simulink model "P4_RaspberryModel_with_DT"  (R2025b)
settings: Solver=daessc  StartTime=0.0  StopTime=Inf  FixedStep=0.01  RelTol=1e-3
PreLoadFcn:
  | % Kalman Filter testing
  | m=0.370;
  | l=0.075; %0.079793%determined by pendulum experiment %former values 0.032, 0.035;
  | lm=l*m; %lm=0.032*0.377
  | r=0.0405;
  | rm=r*m; %rm=0.0405*0.377
  | K=1;
  | 
  | tem=0.2 %initial guess
  | eta=2*lm+rm+(2*m*l^2/r);
  | 
  | A31=(lm+rm)/(tem*eta);
  | A32=9.81*lm/(r*eta);
  | A=[0 1 0 0; 0 -1/tem, 0, 0; 0, 0, 0, 1; 0 A31, A32, 0];
  | B=[0; 1/tem;0;-A31];
model workspace (MAT data in the model file):
  Amp = 1
undefined symbols (not defined in the file): anglerate, DiscIntNeverNeededParam, motor_left, motor_param, motor_right, PosEnc, VelEnc
libraries: simulink x19, raspberrypiCommlib x7, dspstat3 x6, slpidlib x3, sm_lib x3, raspberrypiNetworklib x2, svdutilitieslib x2, SigiLib x2, robotcorelib x1, mspfiltlib x1, nesl_utility x1
(part 1 of 2)
settings Model: SimulationMode=external  NumberOfSteps=10  ExtModeTrigDuration=2  Creator=resjoehr  LastModifiedBy=resjoehr
settings SolverCC: AlgebraicLoopSolver=TrustRegion  PositivePriorityOrder=on
settings OptimizationCC: EnhancedBackFolding=on  PassReuseOutputArgsAs=Individual arguments  ZeroExternalMemoryAtStartup=off  ZeroInternalMemoryAtStartup=off  MaxStackSize=200000  OptimizeBlockOrder=speed  DifferentSizesBufferReuse=on  OptimizationCustomize=off  EfficientTunableParamExpr=on
settings DebuggingCC: ParameterTunabilityLossMsg=error  UnconnectedInputMsg=warning  UnconnectedOutputMsg=warning  UnconnectedLineMsg=warning
settings HardwareCC: ProdBitPerPointer=32.0  ProdBitPerSizeT=32.0  ProdBitPerPtrDiffT=32.0  ProdLargestAtomicInteger=Long  ProdLargestAtomicFloat=Double  ProdWordSize=32.0  ProdLongLongMode=on  ProdHWDeviceType=ARM Compatible->ARM Cortex-A (32-bit)
settings ModelReferenceCC: EnableRefExpFcnMdlSchedulingChecks=on
settings RTWCC: SystemTargetFile=ert.tlc  HardwareBoard=Raspberry Pi  TLCOptions="-aInlineSetEventsForThisBaseRateFcn=TLC_FALSE -aSuppressMultiTaskScheduler=TLC_FALSE  -aRateBasedStepFcn=0"  TemplateMakefile=ert_default_tmf  Toolchain=GNU GCC Embedded Linux  BuildConfiguration=Faster Runs  GPUComputeCapability=3.5  DLArmComputeVersion=19.05  Description=Embedded Coder
settings CodeAppCC: ForceParamTrailComments=on  IgnoreCustomStorageClasses=off  OperatorAnnotations=on  SimulinkDataObjDesc=on  SFDataObjDesc=on  InsertBlockDesc=on
settings ERTTargetCC: ExtModeTransport=2.0  ExtModeStaticAlloc=on  ExtModeMexFile=ext_xcp  ExtModeIntrfLevel=Level2 - Open  InlinedParameterPlacement=Hierarchical  DynamicArrayContainerType=coder::array  SupportVariableSizeSignals=on

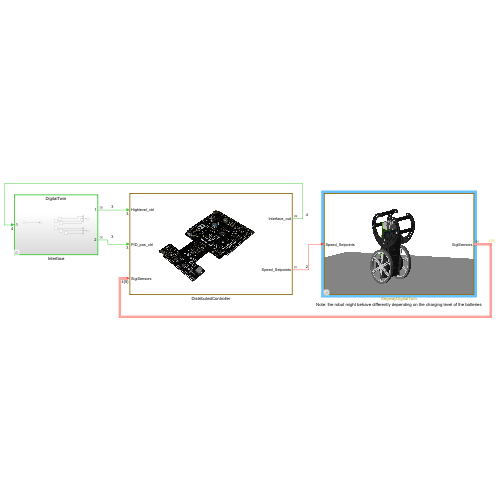
[thumbnail: Simulink's stored preview of the top-level diagram]
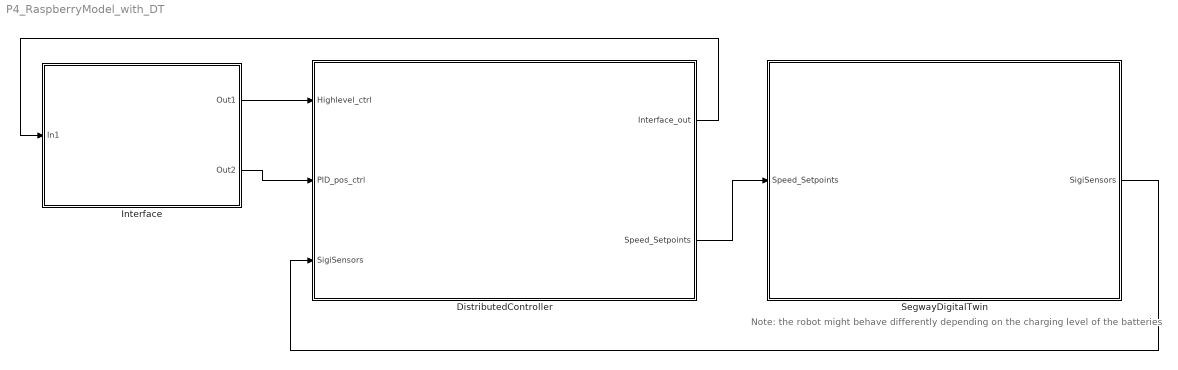
== system P4_RaspberryModel_with_DT ==
  note: Note: the robot might behave differently depending on the charging level of the batteries
  DistributedController : Subsystem
      mask Display: image('leonardo.jpg');
  Interface : Subsystem  Variant=on  VariantControlMode=sim codegen switching
  SegwayDigitalTwin : Subsystem  Variant=on  VariantControlMode=sim codegen switching  VariantControl=SegwayDigitalTwin
      mask Display: image('whole_sigi.jpg');
  wires:
  Interface/1(Out1) -> DistributedController/1(Highlevel_ctrl)
  Interface/2(Out2) -> DistributedController/2(PID_pos_ctrl)
  DistributedController/1(Interface_out) -> Interface/1(In1)
  DistributedController/2(Speed_Setpoints) -> SegwayDigitalTwin/1(Speed_Setpoints)
  SegwayDigitalTwin/1(SigiSensors) -> DistributedController/3(SigiSensors)

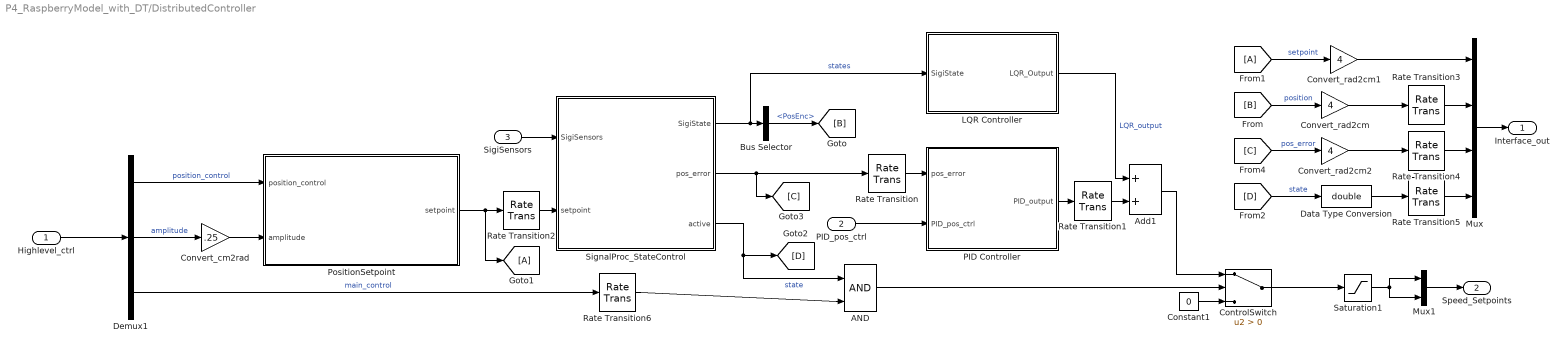
== system P4_RaspberryModel_with_DT/DistributedController ==
  Highlevel_ctrl : Inport  SampleTime=0.1
  PID_pos_ctrl : Inport  Port=2  SampleTime=0.1
  SigiSensors : Inport  Port=3  OutDataTypeStr=Bus: Sensors
  AND : Logic  IconShape=distinctive  AllPortsSameDT=off  OutDataTypeStr=boolean
  Add1 : Sum  OutDataTypeStr=double
  Bus Selector : BusSelector  OutputSignals=PosEnc
  Constant1 : Constant  Value=0  SampleTime=0.01
  ControlSwitch : Switch  Criteria=u2 > Threshold  SaturateOnIntegerOverflow=off  InputSameDT=off
  Convert_cm2rad : Gain  Gain=.25
  Convert_rad2cm : Gain  Gain=4
  Convert_rad2cm1 : Gain  Gain=4
  Convert_rad2cm2 : Gain  Gain=4
  Data Type Conversion : DataTypeConversion  OutDataTypeStr=double  SaturateOnIntegerOverflow=off  RndMeth=Floor
  Demux1 : Demux  Outputs=3
  From1 : From
  Goto1 : Goto
  LQR Controller : Subsystem
  Mux : Mux
  Mux1 : Mux  Inputs=2
  PID Controller : Subsystem
  PositionSetpoint : Subsystem
  Rate Transition{,3..5} (4 alike) : RateTransition  OutPortSampleTime=0.1
  Rate Transition1 : RateTransition  OutPortSampleTime=0.01
  Rate Transition2 : RateTransition  OutPortSampleTime=0.01
  Rate Transition6 : RateTransition  OutPortSampleTime=0.01
  Saturation1 : Saturate  UpperLimit=30  LowerLimit=-30
  SignalProc_StateControl : Subsystem  Variant=on  VariantControlMode=label  LabelModeActiveChoice=SensorFusion
  Interface_out : Outport  SampleTime=0.1
  Speed_Setpoints : Outport  Port=2
  wires:
  Highlevel_ctrl/1 -> Demux1/1
  Demux1/3 -> Rate Transition6/1  "main_control"
  Constant1/1 -> ControlSwitch/3
  AND/1 -> ControlSwitch/2
  Mux1/1 -> Speed_Setpoints/1
  Add1/1 -> ControlSwitch/1
  PID Controller/1(PID_output) -> Rate Transition1/1
  SignalProc_StateControl/3(active) -> [D], AND/1  "state"
  SignalProc_StateControl/1(SigiState) -> Bus Selector/1, LQR Controller/1(SigiState)  "states"
  SigiSensors/1 -> SignalProc_StateControl/1(SigiSensors)
  PID_pos_ctrl/1 -> PID Controller/2(PID_pos_ctrl)
  ControlSwitch/1 -> Saturation1/1
  [C] -> Convert_rad2cm2/1  "pos_error"
  [B] -> Convert_rad2cm/1  "position"
  Mux/1 -> Interface_out/1
  From1/1 -> Convert_rad2cm1/1  "setpoint"
  [D] -> Data Type Conversion/1  "state"
  SignalProc_StateControl/2(pos_error) -> [C], Rate Transition/1
  PositionSetpoint/1(setpoint) -> Goto1/1, Rate Transition2/1
  Demux1/1 -> PositionSetpoint/1(position_control)  "position_control"
  Demux1/2 -> Convert_cm2rad/1  "amplitude"
  Data Type Conversion/1 -> Rate Transition5/1
  Saturation1/1 -> Mux1/1, Mux1/2
  Convert_cm2rad/1 -> PositionSetpoint/2(amplitude)
  Convert_rad2cm/1 -> Rate Transition3/1
  Convert_rad2cm2/1 -> Rate Transition4/1
  Bus Selector/1 -> [B]  "<PosEnc>"
  LQR Controller/1(LQR_Output) -> Add1/1  "LQR_output"
  Rate Transition/1 -> PID Controller/1(pos_error)
  Rate Transition1/1 -> Add1/2
  Convert_rad2cm1/1 -> Mux/1
  Rate Transition3/1 -> Mux/2
  Rate Transition4/1 -> Mux/3
  Rate Transition5/1 -> Mux/4
  Rate Transition6/1 -> AND/2
  Rate Transition2/1 -> SignalProc_StateControl/2(setpoint)

== system P4_RaspberryModel_with_DT/Interface ==
  note: 1) Add Subsystem or Model blocks as valid variant choices.
      | 2) You cannot connect blocks at this level. At simulation, connectivity is automatically
      | determined, based on the active variant and port name matching.
  In1 : Inport
  DigitalTwin : Subsystem  VariantControl=(sim)
  Websocket : Subsystem  VariantControl=(codegen)
  Out1 : Outport
  Out2 : Outport  Port=2

== system P4_RaspberryModel_with_DT/SegwayDigitalTwin ==
  Speed_Setpoints : Inport  OutDataTypeStr=double
  RaspberryImplementation : Subsystem  VariantControl=(codegen)
  SegwayDigitalTwin : Subsystem  VariantControl=(sim)
      mask Display: image('whole_sigi.jpg');
  SigiSensors : Outport  OutDataTypeStr=Bus: Sensors

== system P4_RaspberryModel_with_DT/DistributedController/LQR Controller ==
  SigiState : Inport  OutDataTypeStr=Bus: States
  Bus Selector : BusSelector  OutputSignals=PosEnc,VelEnc,angle,anglerate
  Constant : Constant  Value=1.43  SampleTime=0.01
  Constant1 : Constant  Value=28.6  SampleTime=0.01
  Constant2 : Constant  Value=1.925  SampleTime=0.01
  Gain : Gain  Gain=0
  Product : Product
  Product1 : Product
  Product2 : Product
  Sum : Sum  Inputs=++++
  LQR_Output : Outport
  wires:
  Bus Selector/1 -> Gain/1  "<PosEnc>"
  Sum/1 -> LQR_Output/1
  Bus Selector/4 -> Product2/1  "<anglerate>"
  Bus Selector/3 -> Product1/1  "<angle>"
  Constant/1 -> Product/2
  Constant1/1 -> Product1/2
  Constant2/1 -> Product2/2
  Product/1 -> Sum/2
  Product1/1 -> Sum/3
  Product2/1 -> Sum/4
  Gain/1 -> Sum/1
  SigiState/1 -> Bus Selector/1
  Bus Selector/2 -> Product/1  "<VelEnc>"

== system P4_RaspberryModel_with_DT/DistributedController/PID Controller ==
  pos_error : Inport
  PID_pos_ctrl : Inport  Port=2
  Demux2 : Demux  Outputs=3
  Filter : Constant  Value=10  SampleTime=0.1
  Gain : Gain  Gain=-1
  Gain1 : Gain  Gain=-1
  Gain2 : Gain  Gain=-1
  Position Controller1 : slpidlib/PID Controller  Controller=PID  Form=Parallel  TimeDomain=Discrete-time  UseExternalTs=off  SampleTime=0.1  IntegratorMethod=Forward Euler  FilterMethod=Forward Euler  ControllerParametersSource=external  P=-0.3  I=0  UseKiTs=off  D=0.1  UseExternalDerivativeSource=off  N=10  UseFilter=on  TunerSelectOption=Transfer Function Based (PID Tuner App)  InitialConditionSource=internal  InitialConditionForIntegrator=0  InitialConditionForFilter=0  DifferentiatorICPrevScaledInput=0  ExternalReset=none  TrackingMode=off  Kt=1  LimitOutput=on  SatLimitsSource=internal  UpperSaturationLimit=20  LowerSaturationLimit=-20  LinearizeAsGain=on  AntiWindupMode=none  Kb=1  LimitIntegrator=off  UpperIntegratorSaturationLimit=inf  LowerIntegratorSaturationLimit=-inf  POutMin=[]  POutMax=[]  IOutMin=[]  IOutMax=[]  DOutMin=[]  DOutMax=[]  NOutMin=[]  NOutMax=[]  SumOutMin=[]  SumOutMax=[]  SaturationOutMin=[]  SaturationOutMax=[]  PParamMin=[]  PParamMax=[]  IParamMin=[]  IParamMax=[]  DParamMin=[]  DParamMax=[]  NParamMin=[]  NParamMax=[]  KbParamMin=[]  KbParamMax=[]  KtParamMin=[]  KtParamMax=[]  KbOutMin=[]  KbOutMax=[]  KtOutMin=[]  KtOutMax=[]  IntegratorOutMin=[]  IntegratorOutMax=[]  FilterOutMin=[]  FilterOutMax=[]  SumI1OutMin=[]  SumI1OutMax=[]  SumI2OutMin=[]  SumI2OutMax=[]  SumI3OutMin=[]  SumI3OutMax=[]  SumI4OutMin=[]  SumI4OutMax=[]  SumDOutMin=[]  SumDOutMax=[]  DifferentiatorOutMin=[]  DifferentiatorOutMax=[]  FilterDiffOutCoefMin=[]  FilterDiffOutCoefMax=[]  ReciprocalOutMin=[]  ReciprocalOutMax=[]  SumDenOutMin=[]  SumDenOutMax=[]  SumNumOutMin=[]  SumNumOutMax=[]  DivideOutMin=[]  DivideOutMax=[]  UdiffTsProdOutMin=[]  UdiffTsProdOutMax=[]  NTsProdOutMin=[]  NTsProdOutMax=[]  UintegralTsProdOutMin=[]  UintegralTsProdOutMax=[]  UngainTsProdOutMin=[]  UngainTsProdOutMax=[]  ClampingZeroOutDataTypeStr=Inherit: Inherit via back propagation  ClampingZeroOutMin=[]  ClampingZeroOutMax=[]  FilterDenConstantOutDataTypeStr=Inherit: Inherit via back propagation  FilterDenConstantOutMin=[]  FilterDenConstantOutMax=[]  PCopyOutDataTypeStr=Inherit: Inherit via back propagation  PCopyOutMin=[]  PCopyOutMax=[]  NCopyOutDataTypeStr=Inherit: Inherit via back propagation  NCopyOutMin=[]  NCopyOutMax=[]  IntegratorContinuousStateAttributes=''  IntegratorStateMustResolveToSignalObject=off  IntegratorRTWStateStorageClass=Auto  FilterContinuousStateAttributes=''  FilterStateMustResolveToSignalObject=off  FilterRTWStateStorageClass=Auto  ParallelPVariant=ExternalParameters  IdealPVariant=Disabled  IVariant=ExternalParameters  DVariant=ExternalParameters  IntegratorVariant=Discrete  SatVariant=Enabled  AWVariant=Passthrough  PCopyVariant=Disabled  TRVariant=Disabled  FdbkBlocksVariant=Forward  IdealPFdbkVariant=Disabled  SatFdbkVariant=Disabled  DerivativeFilterVariant=ForwardEulerFilter  NVariant=ExternalParameters  NCopyVariant=Disabled  FilterICVariant=InternalICsFilter  IntegratorICVariant=InternalICs  ExternalResetVariant=Disabled  TRSumVariant=Passthrough  SumFdbkVariant=Disabled  SumVariant=Sum_PID  TsampFilterVariant=InternalTs  TsampNgainVariant=Passthrough  TsampIntegralVariant=Disabled_SignalSpec  ExternalSaturationOutDataTypeStr=Inherit: Same as second input  DerivativeSourceVariant=ErrorSignal  PreIntVariant=InternalPreInt
  PID_output : Outport
  wires:
  Demux2/1 -> Gain/1
  Gain2/1 -> Position Controller1/4
  Gain/1 -> Position Controller1/2
  Filter/1 -> Position Controller1/5
  Demux2/3 -> Gain2/1
  Gain1/1 -> Position Controller1/3
  Demux2/2 -> Gain1/1
  PID_pos_ctrl/1 -> Demux2/1
  pos_error/1 -> Position Controller1/1  "setpoint"
  Position Controller1/1 -> PID_output/1

== system P4_RaspberryModel_with_DT/DistributedController/PositionSetpoint ==
  note: Position Setpoint
  position_control : Inport
  amplitude : Inport  Port=2
  Add3 : Sum  Inputs=+-
  Gain : Gain  Gain=0
  Gain5 : Gain
  Product1 : Product  Inputs=3
  Pulse Generator1 : DiscretePulseGenerator  Period=200  PulseWidth=100  PhaseDelay=100  SampleTime=0.1
  setpoint : Outport
  wires:
  Product1/1 -> Gain5/1  "setpoint"
  Gain/1 -> Add3/2
  Gain5/1 -> Add3/1
  amplitude/1 -> Product1/2, Gain/1
  Pulse Generator1/1 -> Product1/3
  Add3/1 -> setpoint/1  "setpoint"
  position_control/1 -> Product1/1

== system P4_RaspberryModel_with_DT/DistributedController/SignalProc_StateControl ==
  note: 1) Add Subsystem or Model blocks as valid variant choices.
      | 2) You cannot connect blocks at this level. At simulation, connectivity is automatically
      | determined, based on the active variant and port name matching.
  SigiSensors : Inport  OutDataTypeStr=Bus: Sensors
  setpoint : Inport  Port=2
  ClassicalCalibration : Subsystem  VariantControl=ClassicalCalibration
  SensorFusion : Subsystem  VariantControl=SensorFusion
  SigiState : Outport  OutDataTypeStr=Bus: States
  pos_error : Outport  Port=2
  active : Outport  Port=3

== system P4_RaspberryModel_with_DT/Interface/DigitalTwin ==
  In1 : Inport  OutDataTypeStr=double
  Constant : Constant  Value=0  SampleTime=0.1
  Constant1 : Constant  Value=0  SampleTime=0.1
  Constant2 : Constant  Value=0.5  SampleTime=0.1
  Constant3 : Constant  SampleTime=0.1
  Constant4 : Constant  SampleTime=0.1
  Constant5 : Constant  Value=10  SampleTime=0.1
  Mux2 : Mux  Inputs=3
  Mux3 : Mux  Inputs=3
  Terminator : Terminator
  Out1 : Outport
  Out2 : Outport  Port=2
  wires:
  In1/1 -> Terminator/1
  Constant5/1 -> Mux2/2  "amplitude"
  Constant3/1 -> Mux2/3  "main control"
  Constant4/1 -> Mux2/1  "enable_pos_control"
  Mux2/1 -> Out1/1
  Constant2/1 -> Mux3/1  "p-gain"
  Mux3/1 -> Out2/1
  Constant1/1 -> Mux3/2  "i-gain"
  Constant/1 -> Mux3/3  "d-gain"

== system P4_RaspberryModel_with_DT/Interface/Websocket ==
  In1 : Inport
  Demux : Demux
  FromWebSocket : Subsystem
  Websocket publish : raspberrypiNetworklib/WebSocket publish  UniqueBlockID=webPub 1  IPAddress=192.168.43.245  Port=9000  NumberOfSignals=4  webSocketId=P4_RaspberryModel_with_DT/Interface/Websocket/Websocket_publish  BlockPlatform=RASPBERRYPI
  Out1 : Outport
  Out2 : Outport  Port=2
  wires:
  In1/1 -> Demux/1
  Demux/1 -> Websocket publish/1
  Demux/2 -> Websocket publish/2
  Demux/3 -> Websocket publish/3
  Demux/4 -> Websocket publish/4
  FromWebSocket/2(Out2) -> Out2/1
  FromWebSocket/1(Out1) -> Out1/1

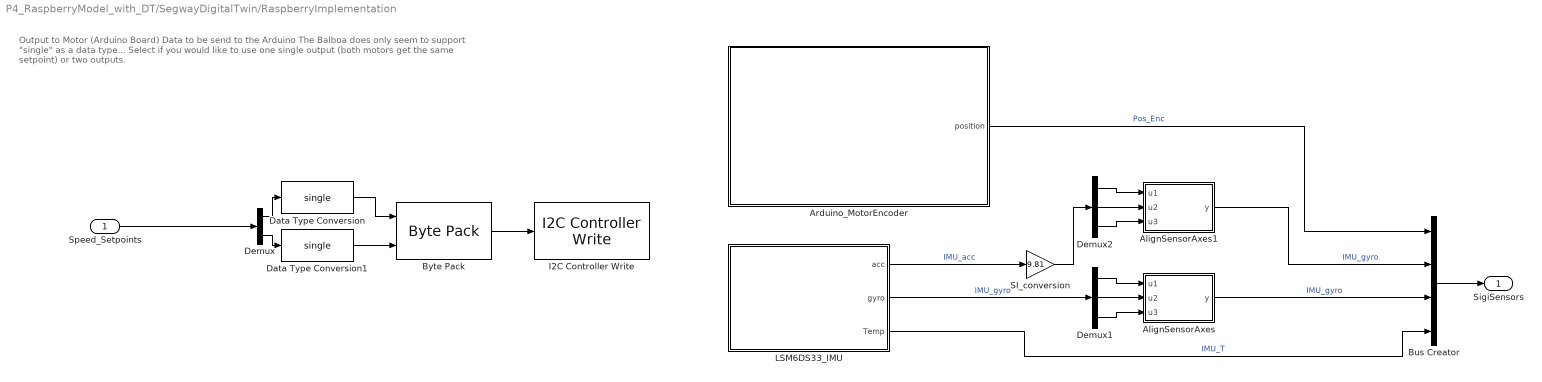
== system P4_RaspberryModel_with_DT/SegwayDigitalTwin/RaspberryImplementation ==
  note: Output to Motor (Arduino Board)
      | Data to be send to the Arduino
      | The Balboa does only seem to support "single" as a data type...
      | Select if you would like to use one single output (both motors get the same setpoint)
      | or two outputs.
  Speed_Setpoints : Inport  OutDataTypeStr=double
  AlignSensorAxes : MATLAB Function  TreatAsAtomicUnit=on
  AlignSensorAxes1 : MATLAB Function  TreatAsAtomicUnit=on
  Arduino_MotorEncoder : Subsystem
  Bus Creator : BusCreator  Inputs=4  OutDataTypeStr=Bus: Sensors
      settings: InheritFromInputs=off
  Byte Pack : svdutilitieslib/Byte Pack  maskPackedDataType=uint8  datatypes={'single','single'}  byteAlign=1  blockPlatform=arduinoert
  Data Type Conversion : DataTypeConversion  OutDataTypeStr=single  SaturateOnIntegerOverflow=off  RndMeth=Floor
  Data Type Conversion1 : DataTypeConversion  OutDataTypeStr=single  SaturateOnIntegerOverflow=off  RndMeth=Floor
  Demux : Demux  Outputs=2
  Demux1 : Demux  Outputs=3
  Demux2 : Demux  Outputs=3
  I2C Controller Write : raspberrypiCommlib/I2C Controller Write  BoardProperty=Pi 3 Model B+  I2CModule=1  Mode=Master  SlaveAddress=10  SlaveByteOrder=BigEndian  Direction=Transmitter  RegisterAddressMode=off  RegisterAddress=0  SlaveDataType=uint8  DataLength=1  NoAck=off  RepeatedStart=off  OutputStatus=off
  LSM6DS33_IMU : Subsystem
  SI_conversion : Gain  Gain=9.81
  SigiSensors : Outport  OutDataTypeStr=Bus: Sensors
  wires:
  Demux/1 -> Data Type Conversion/1
  Demux/2 -> Data Type Conversion1/1
  Speed_Setpoints/1 -> Demux/1
  Data Type Conversion/1 -> Byte Pack/1
  Byte Pack/1 -> I2C Controller Write/1
  Data Type Conversion1/1 -> Byte Pack/2
  LSM6DS33_IMU/1(acc) -> SI_conversion/1  "IMU_acc"
  LSM6DS33_IMU/2(gyro) -> Demux1/1  "IMU_gyro"
  LSM6DS33_IMU/3(Temp) -> Bus Creator/4  "IMU_T"
  Arduino_MotorEncoder/1(position) -> Bus Creator/1  "Pos_Enc"
  Bus Creator/1 -> SigiSensors/1
  Demux1/2 -> AlignSensorAxes/2(u2)
  Demux1/1 -> AlignSensorAxes/1(u1)
  Demux1/3 -> AlignSensorAxes/3(u3)
  AlignSensorAxes/1(y) -> Bus Creator/3  "IMU_gyro"
  Demux2/3 -> AlignSensorAxes1/3(u3)
  Demux2/1 -> AlignSensorAxes1/1(u1)
  Demux2/2 -> AlignSensorAxes1/2(u2)
  SI_conversion/1 -> Demux2/1
  AlignSensorAxes1/1(y) -> Bus Creator/2  "IMU_gyro"

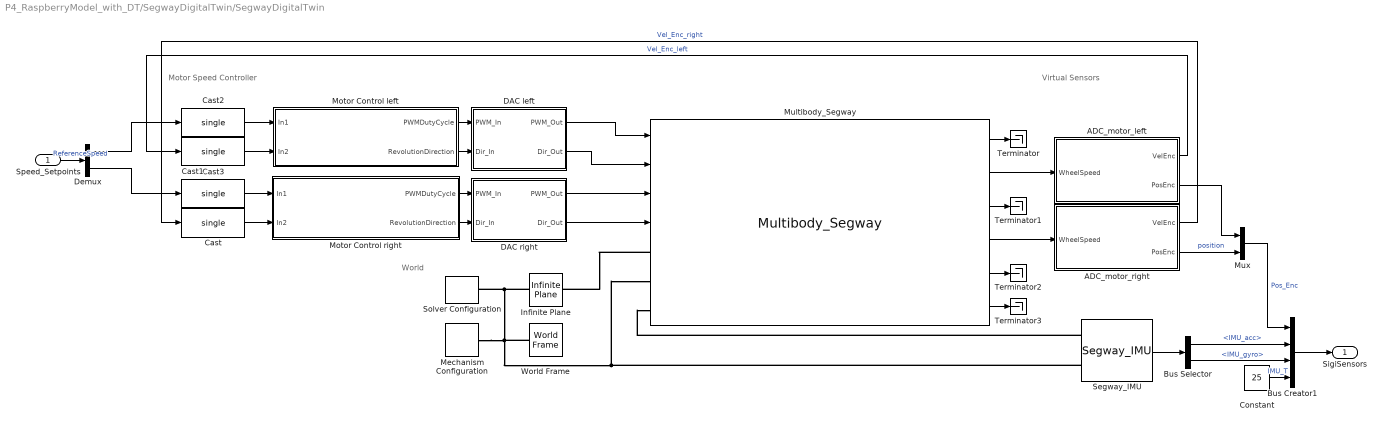
== system P4_RaspberryModel_with_DT/SegwayDigitalTwin/SegwayDigitalTwin ==
  note: Motor Speed Controller
  note: World
  note: Virtual Sensors
  Speed_Setpoints : Inport  OutDataTypeStr=double  PortDimensions=2  SampleTime=[0.01,0]
  ADC_motor_left : Subsystem
  ADC_motor_right : Subsystem
  Bus Creator1 : BusCreator  Inputs=4  OutDataTypeStr=Bus: Sensors
      settings: InheritFromInputs=off
  Bus Selector : BusSelector  OutputSignals=IMU_acc,IMU_gyro
  Cast{,1..3} (4 alike) : DataTypeConversion  OutDataTypeStr=single  SaturateOnIntegerOverflow=off  RndMeth=Floor
  Constant : Constant  Value=25  SampleTime=0.01
  DAC left : Subsystem
      settings: PortSchema="{\"entries\":[{\"content\":{\"sides\":[{\"content\":{},\"type\":\"ConnectorPlacement.EquallySpacedRectSide\",\"uuid\":\"2a048367-e2f0-4bba-953c-ae910e274789\"},{\"content\":{\"side\":\"RIGHT\"},\"type\":\"ConnectorPlacement.EquallySpacedRectSide\",\"uuid\":\"7ccde743-fca2-43e4-b0c2-cd13b64bc8b1\"},{\"content\":{\"connectorIds\":[\"In1\",\"In2\"],\"side\":\"TOP\"},\"type\":\"ConnectorPlacement.EquallySpacedRectSide\",\"uuid\":\"3ce48c05-91da-4625-95ec-e1126e256571\"},{\"content\":{\"connectorIds\":[\"Out1\",\"Out2\"],\"side\":\"BOTTOM\"},\"type\":\"ConnectorPlacement.EquallySpacedRectSide\",\"uuid\":\"d3272110-62c8-461d-b270-1e960017d7b6\"}]},\"type\":\"ConnectorPlacement.EquallySpacedConnector\",\"uuid\":\"12bb8b59-2cea-4810-9f9c-b5dd2504e4e2\"}],\"packageUris\":[\"http://schema.mathworks.com/mf0/Connector/R2020b\"],\"version\":\"1.0\"}"
  DAC right : Subsystem
      settings: PortSchema="{\"entries\":[{\"content\":{\"sides\":[{\"content\":{},\"type\":\"ConnectorPlacement.EquallySpacedRectSide\",\"uuid\":\"2a048367-e2f0-4bba-953c-ae910e274789\"},{\"content\":{\"side\":\"RIGHT\"},\"type\":\"ConnectorPlacement.EquallySpacedRectSide\",\"uuid\":\"7ccde743-fca2-43e4-b0c2-cd13b64bc8b1\"},{\"content\":{\"connectorIds\":[\"In1\",\"In2\"],\"side\":\"TOP\"},\"type\":\"ConnectorPlacement.EquallySpacedRectSide\",\"uuid\":\"3ce48c05-91da-4625-95ec-e1126e256571\"},{\"content\":{\"connectorIds\":[\"Out1\",\"Out2\"],\"side\":\"BOTTOM\"},\"type\":\"ConnectorPlacement.EquallySpacedRectSide\",\"uuid\":\"d3272110-62c8-461d-b270-1e960017d7b6\"}]},\"type\":\"ConnectorPlacement.EquallySpacedConnector\",\"uuid\":\"12bb8b59-2cea-4810-9f9c-b5dd2504e4e2\"}],\"packageUris\":[\"http://schema.mathworks.com/mf0/Connector/R2020b\"],\"version\":\"1.0\"}"
  Demux : Demux  Outputs=2
  Infinite Plane : sm_lib/Curves and Surfaces/Infinite Plane  GraphicType=Rectangle  GraphicPlaneWidth=1  GraphicPlaneWidthUnits=m  GraphicPlaneHeight=1  GraphicPlaneHeightUnits=m  GraphicVisPropType=SimpleVisualProperties  GraphicDiffuseColor=[0.5 0.5 0.5]  GraphicOpacity=0.25  GraphicSpecularColor=[0.5 0.5 0.5 1.0]  GraphicAmbientColor=[0.15 0.15 0.15 1.0]  GraphicEmissiveColor=[0.0 0.0 0.0 1.0]  GraphicShininess=75
  Mechanism Configuration : sm_lib/Utilities/Mechanism Configuration  UniformGravity=Constant  GravityVector=[0 0 -9.80665]  GravityVectorUnits=m/s^2  LinearizationDelta=0.001  JointModeTransitionNonlinearIterations=2
  Motor Control left : Subsystem
      settings: PortSchema="{\"entries\":[{\"content\":{\"sides\":[{\"content\":{\"connectorIds\":[\"Out1\",\"Out2\"]},\"type\":\"ConnectorPlacement.EquallySpacedRectSide\",\"uuid\":\"2a048367-e2f0-4bba-953c-ae910e274789\"},{\"content\":{\"connectorIds\":[\"In1\",\"In2\"],\"side\":\"RIGHT\"},\"type\":\"ConnectorPlacement.EquallySpacedRectSide\",\"uuid\":\"7ccde743-fca2-43e4-b0c2-cd13b64bc8b1\"},{\"content\":{\"side\":\"TOP\"},\"type\":\"ConnectorPlacement.EquallySpacedRectSide\",\"uuid\":\"3ce48c05-91da-4625-95ec-e1126e256571\"},{\"content\":{\"side\":\"BOTTOM\"},\"type\":\"ConnectorPlacement.EquallySpacedRectSide\",\"uuid\":\"43d129b0-e351-40fa-8830-2340ea4b3634\"}]},\"type\":\"ConnectorPlacement.EquallySpacedConnector\",\"uuid\":\"12bb8b59-2cea-4810-9f9c-b5dd2504e4e2\"}],\"packageUris\":[\"http://schema.mathworks.com/mf0/Connector/R2020b\"],\"version\":\"1.0\"}"
  Motor Control right : Subsystem
  Multibody_Segway : SigiLib/Multibody_Segway  Parameter3=0  Parameter2=0
  Mux : Mux  Inputs=2
  Segway_IMU : SigiLib/Segway_IMU  SystemSampleTime=-1  VariantActivationTime=update diagram  EmptyChoice=off  PassThrough=off  PassThroughVariantControl=(default)  EmptyChoiceVariantControl=(default)  AllowFlexibleInterface=on  Latency=0  AutoFrameSizeCalculation=off
  Solver Configuration : nesl_utility/Solver Configuration  PhysicalDomain=network_engine_domain  SubClassName=solver  LeftPortType=input  RightPortType=generic  Tones=[]  Harmonics=[]  SimulateNoise=off  Profile=off  UseLocalSampling=off  EnableSwitchedLinearOptims=on  FrequencyDomain=off  UseCCode=off  RelTol=0.001  AbsTol=1e-06  MinStep=1e-09  ToWorkspace=off  RevertToSquareIcSolve=off  NumHomotopyIterations=100  PhasorMode=off  PhasorModeNumHarmonics=1  ConsistencySolver=NEWTON_FTOL  IndexReductionMethod=DerivativeReplacement  DoDC=off  ResidualTolerance=1e-09  ConsistencyTolSource=GLOBAL  ConsistencyAbsTol=0.001  ConsistencyRelTol=0.001  ConsistencyTolFactor=0.001  UseLocalSolver=off  LocalSolverChoice=NE_BACKWARD_EULER_ADVANCER  ResolveIndetEquations=on  FunctionEvalNumThread=1  LocalSolverSampleTime=0.001  DoFixedCost=off  MaxNonlinIter=3  MaxModeIter=2  ComputeImpulses=off  ImpulseIterations=2  LinearAlgebra=Sparse  LinearAlgebraNumThread=0  EquationFormulation=NE_TIME_EF  DelaysMemoryBudget=1024  AutomaticFiltering=on  FilteringTimeConstant=0.001  PartitionStorageMethod=AS_NEEDED  PartitionMemoryBudget=1024  PartitionMethod=FAST  MultibodyUseLocalSolver=off  MultibodyLocalSolverChoice=ODE1  MultibodyLocalSolverSampleTime=0.001
  Terminator{,1..3} (4 alike) : Terminator
  World Frame : sm_lib/Frames and Transforms/World Frame
  SigiSensors : Outport  OutDataTypeStr=Bus: Sensors
  wires:
  DAC right/1(PWM_Out) -> Multibody_Segway/3
  Cast1/1 -> Motor Control right/1(In1)
  Motor Control right/2(RevolutionDirection) -> DAC right/2(Dir_In)
  Cast/1 -> Motor Control right/2(In2)
  Segway_IMU/1 -> Bus Selector/1
  DAC right/2(Dir_Out) -> Multibody_Segway/4
  Speed_Setpoints/1 -> Demux/1  "ReferenceSpeed"
  ADC_motor_right/1(VelEnc) -> Cast/1  "Vel_Enc_right"
  Motor Control right/1(PWMDutyCycle) -> DAC right/1(PWM_In)
  ADC_motor_right/2(PosEnc) -> Mux/2  "position"
  Cast2/1 -> Motor Control left/1(In1)
  Motor Control left/1(PWMDutyCycle) -> DAC left/1(PWM_In)
  Motor Control left/2(RevolutionDirection) -> DAC left/2(Dir_In)
  DAC left/2(Dir_Out) -> Multibody_Segway/2
  DAC left/1(PWM_Out) -> Multibody_Segway/1
  ADC_motor_left/1(VelEnc) -> Cast3/1  "Vel_Enc_left"
  Cast3/1 -> Motor Control left/2(In2)
  ADC_motor_left/2(PosEnc) -> Mux/1
  Demux/2 -> Cast1/1
  Demux/1 -> Cast2/1
  Mux/1 -> Bus Creator1/1  "Pos_Enc"
  Constant/1 -> Bus Creator1/4  "IMU_T"
  Bus Creator1/1 -> SigiSensors/1
  Bus Selector/1 -> Bus Creator1/2  "<IMU_acc>"
  Bus Selector/2 -> Bus Creator1/3  "<IMU_gyro>"
  Multibody_Segway/2 -> ADC_motor_left/1(WheelSpeed)
  Multibody_Segway/4 -> ADC_motor_right/1(WheelSpeed)
  Multibody_Segway/1 -> Terminator/1
  Multibody_Segway/3 -> Terminator1/1
  Multibody_Segway/5 -> Terminator2/1
  Multibody_Segway/6 -> Terminator3/1
  connections:
  Multibody_Segway/LConn1 -- Infinite Plane/RConn1
  Infinite Plane/LConn1 -- Segway_IMU/LConn2 -- Multibody_Segway/LConn2 -- World Frame/RConn1 -- Mechanism Configuration/RConn1 -- Solver Configuration/RConn1
  Segway_IMU/LConn1 -- Multibody_Segway/LConn3

== system P4_RaspberryModel_with_DT/DistributedController/SignalProc_StateControl/ClassicalCalibration ==
  SigiSensors : Inport  OutDataTypeStr=Bus: Sensors
  setpoint : Inport  Port=2
  SensorProcessing : Subsystem
  Statemachine_Old : Subsystem
  SigiState : Outport  OutDataTypeStr=Bus: States
  pos_error : Outport  Port=2
  active : Outport  Port=3
  wires:
  SensorProcessing/1(Out1) -> Statemachine_Old/1(In1)
  Statemachine_Old/1(SigiState) -> SigiState/1
  SigiSensors/1 -> SensorProcessing/1(In1)
  setpoint/1 -> Statemachine_Old/2(setpoint)
  Statemachine_Old/2(pos_error) -> pos_error/1
  Statemachine_Old/3(active) -> active/1

== system P4_RaspberryModel_with_DT/DistributedController/SignalProc_StateControl/SensorFusion ==
  SigiSensors : Inport  OutDataTypeStr=Bus: Sensors
  setpoint : Inport  Port=2
  SensorFusion : Subsystem
  Statemachine : Subsystem
  SigiState : Outport  OutDataTypeStr=Bus: States
  pos_error : Outport  Port=2
  active : Outport  Port=3
  wires:
  SensorFusion/1(Out1) -> Statemachine/1(sensors_raw)
  SigiSensors/1 -> SensorFusion/1(In1)
  Statemachine/1(SigiState) -> SigiState/1  "states"
  Statemachine/2(pos_error) -> pos_error/1
  Statemachine/3(active) -> active/1  "state"
  setpoint/1 -> Statemachine/2(setpoint)

== system P4_RaspberryModel_with_DT/Interface/Websocket/FromWebSocket ==
  Demux : Demux  Outputs=6
  Mux : Mux  Inputs=6
  Mux2 : Mux  Inputs=3
  Mux3 : Mux  Inputs=3
  Switch : Switch  Criteria=u2 > Threshold  SaturateOnIntegerOverflow=off  InputSameDT=off
  Unit Delay : UnitDelay  InitialCondition=[0, 0, 1, -0.8, 0, 0]  SampleTime=-1  HasFrameUpgradeWarning=on
  WebSocket subscribe : raspberrypiNetworklib/WebSocket subscribe  IPAddress=192.168.43.245  Port=9000  OutputCfg=Mask Dialog  numSignals=6  Dsize1=1  Dtype1=double  Dsize2=1  Dtype2=double  Dsize3=1  Dtype3=double  Dsize4=1  Dtype4=double  Dsize5=1  Dtype5=double  Dsize6=1  Dtype6=double  Dsize7=1  Dtype7=double  Dsize8=1  Dtype8=double  Dsize9=1  Dtype9=double  Dsize10=1  Dtype10=double  Sampletime=0.1  NumberOfSignals=6  webSocketId=P4_RaspberryModel_with_DT/Interface/Websocket/FromWebSocket/WebSocket_subscribe  BlockPlatform=RASPBERRYPI
  Out1 : Outport  SampleTime=0.1
  Out2 : Outport  Port=2  SampleTime=0.1
  wires:
  WebSocket subscribe/2 -> Mux/1
  Switch/1 -> Demux/1, Unit Delay/1
  WebSocket subscribe/5 -> Mux/4
  Demux/4 -> Mux3/1  "p-gain"
  WebSocket subscribe/7 -> Mux/6
  WebSocket subscribe/3 -> Mux/2
  Demux/5 -> Mux3/2  "i-gain"
  Demux/6 -> Mux3/3  "d-gain"
  WebSocket subscribe/6 -> Mux/5
  Mux/1 -> Switch/1
  WebSocket subscribe/4 -> Mux/3
  WebSocket subscribe/1 -> Switch/2
  Demux/2 -> Mux2/1  "enable_pos_control"
  Demux/3 -> Mux2/2  "amplitude"
  Unit Delay/1 -> Switch/3
  Demux/1 -> Mux2/3  "main control"
  Mux2/1 -> Out1/1
  Mux3/1 -> Out2/1

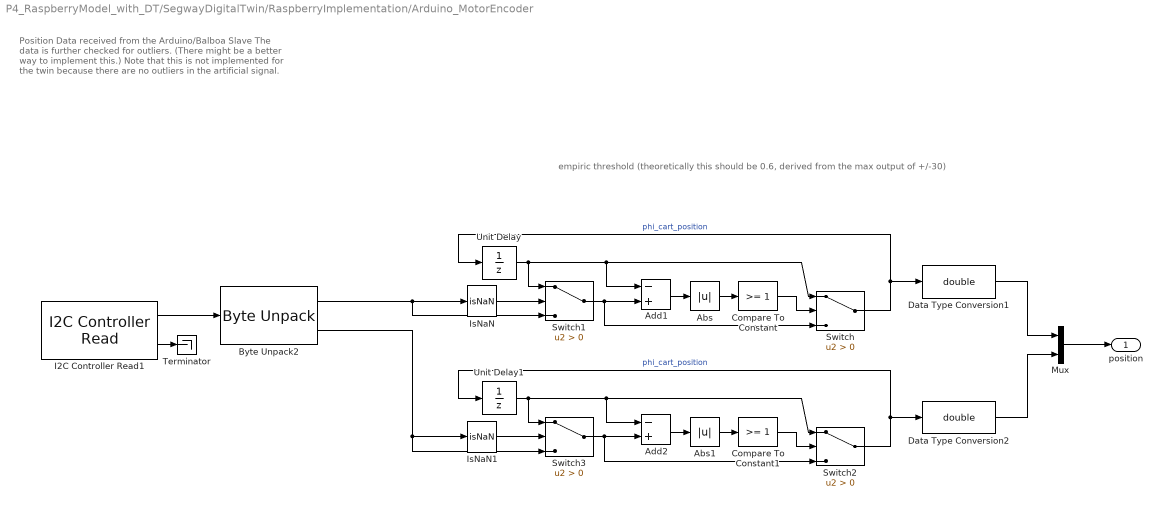
== system P4_RaspberryModel_with_DT/SegwayDigitalTwin/RaspberryImplementation/Arduino_MotorEncoder ==
  note: empiric threshold (theoretically this should be 0.6, derived from the max output of +/-30)
  note: Position Data received from the Arduino/Balboa Slave
      | The data is further checked for outliers.
      | (There might be a better way to implement this.)
      | Note that this is not implemented for the twin because there are no outliers in the artificial signal.
  Abs : Abs  SaturateOnIntegerOverflow=off
  Abs1 : Abs  SaturateOnIntegerOverflow=off
  Add1 : Sum  Inputs=-+
  Add2 : Sum  Inputs=-+
  Byte Unpack2 : svdutilitieslib/Byte Unpack  dimensions={[1],[1]}  datatypes={'single','single'}  byteAlign=1  blockPlatform=arduinoert
  Compare To Constant : simulink/Logic and Bit Operations/Compare To Constant  relop=>=  const=1  OutDataTypeStr=boolean
  Compare To Constant1 : simulink/Logic and Bit Operations/Compare To Constant  relop=>=  const=1  OutDataTypeStr=boolean
  Data Type Conversion1 : DataTypeConversion  OutDataTypeStr=double  SaturateOnIntegerOverflow=off  RndMeth=Floor
  Data Type Conversion2 : DataTypeConversion  OutDataTypeStr=double  SaturateOnIntegerOverflow=off  RndMeth=Floor
  I2C Controller Read1 : raspberrypiCommlib/I2C Controller Read  BoardProperty=Pi 3 Model B+  I2CModule=1  Mode=Master  SlaveAddress=10  SlaveByteOrder=BigEndian  Direction=Receiver  RegisterAddressMode=off  RegisterAddress=0  SlaveDataType=uint8  DataLength=8  NoAck=off  RepeatedStart=off  OutputStatus=on  SampleTime=0.01
  IsNaN : RelationalOperator  Operator=isNaN  OutDataTypeStr=boolean  RndMeth=Simplest  InputSameDT=off
  IsNaN1 : RelationalOperator  Operator=isNaN  OutDataTypeStr=boolean  RndMeth=Simplest  InputSameDT=off
  Mux : Mux  Inputs=2
  Switch{,1..3} (4 alike) : Switch  Criteria=u2 > Threshold  SaturateOnIntegerOverflow=off  InputSameDT=off
  Terminator : Terminator
  Unit Delay : UnitDelay  SampleTime=-1  HasFrameUpgradeWarning=on
  Unit Delay1 : UnitDelay  SampleTime=-1  HasFrameUpgradeWarning=on
  position : Outport  PortDimensions=2
  wires:
  IsNaN/1 -> Switch1/2
  Compare To Constant/1 -> Switch/2
  Byte Unpack2/1 -> Switch1/3, IsNaN/1
  Unit Delay/1 -> Switch/1, Add1/1, Switch1/1
  Switch1/1 -> Add1/2, Switch/3
  Switch/1 -> Unit Delay/1, Data Type Conversion1/1  "phi_cart_position"
  Abs/1 -> Compare To Constant/1
  Add1/1 -> Abs/1
  I2C Controller Read1/1 -> Byte Unpack2/1
  I2C Controller Read1/2 -> Terminator/1
  Data Type Conversion1/1 -> Mux/1
  Data Type Conversion2/1 -> Mux/2
  Byte Unpack2/2 -> Switch3/3, IsNaN1/1
  Abs1/1 -> Compare To Constant1/1
  Add2/1 -> Abs1/1
  Unit Delay1/1 -> Switch2/1, Add2/1, Switch3/1
  IsNaN1/1 -> Switch3/2
  Switch2/1 -> Unit Delay1/1, Data Type Conversion2/1  "phi_cart_position"
  Compare To Constant1/1 -> Switch2/2
  Switch3/1 -> Add2/2, Switch2/3
  Mux/1 -> position/1

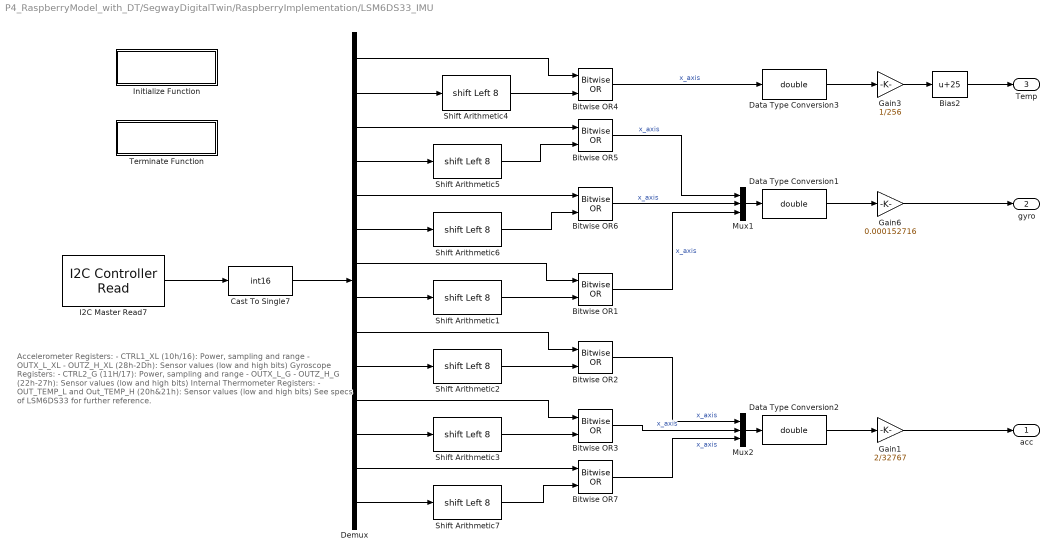
== system P4_RaspberryModel_with_DT/SegwayDigitalTwin/RaspberryImplementation/LSM6DS33_IMU ==
  note: Accelerometer Registers:
      | - CTRL1_XL (10h/16): Power, sampling and range
      | - OUTX_L_XL - OUTZ_H_XL (28h-2Dh): Sensor values (low and high bits)
      |
      | Gyroscope Registers:
      | - CTRL2_G (11H/17): Power, sampling and range
      | - OUTX_L_G - OUTZ_H_G (22h-27h): Sensor values (low and high bits)
      |
      | Internal Thermometer Registers:
      | - OUT_TEMP_L and Out_TEMP_H (20h&21h): Sensor values (low and high bits)
      |
      | See specs of LSM6DS33 for further reference.
  Bias2 : Bias  Bias=25  SaturateOnIntegerOverflow=off
  Bitwise OR{1..7} (7 alike) : simulink/Logic and Bit Operations/Bitwise Operator  logicop=OR  UseBitMask=off  NumInputPorts=2  BitMask=bin2dec('11011001')  BitMaskRealWorld=Stored Integer
  Cast To Single7 : DataTypeConversion  OutDataTypeStr=int16  SaturateOnIntegerOverflow=off  RndMeth=Floor
  Data Type Conversion1 : DataTypeConversion  OutDataTypeStr=double  SaturateOnIntegerOverflow=off  RndMeth=Floor
  Data Type Conversion2 : DataTypeConversion  OutDataTypeStr=double  SaturateOnIntegerOverflow=off  RndMeth=Floor
  Data Type Conversion3 : DataTypeConversion  OutDataTypeStr=double  SaturateOnIntegerOverflow=off  RndMeth=Floor
  Demux : Demux  Outputs=14
  Gain1 : Gain  Gain=2/32767
  Gain3 : Gain  Gain=1/256
  Gain6 : Gain  Gain=0.000152716
  I2C Master Read7 : raspberrypiCommlib/I2C Controller Read  BoardProperty=Pi 3 Model B+  I2CModule=1  Mode=Master  SlaveAddress=107  SlaveByteOrder=BigEndian  Direction=Receiver  RegisterAddressMode=on  RegisterAddress=hex2dec('20')  SlaveDataType=uint8  DataLength=14  NoAck=off  RepeatedStart=off  OutputStatus=off  SampleTime=0.01
  Initialize Function : Subsystem  TreatAsAtomicUnit=on
  Mux1 : Mux  Inputs=3
  Mux2 : Mux  Inputs=3
  Shift Arithmetic{1..7} (7 alike) : ArithShift  BitShiftNumber=8  BitShiftDirection=Left
  Terminate Function : Subsystem  TreatAsAtomicUnit=on
  acc : Outport
  gyro : Outport  Port=2
  Temp : Outport  Port=3
  wires:
  Bitwise OR7/1 -> Mux2/3  "x_axis"
  Bitwise OR1/1 -> Mux1/3  "x_axis"
  Shift Arithmetic2/1 -> Bitwise OR2/2
  Shift Arithmetic1/1 -> Bitwise OR1/2
  Demux/7 -> Bitwise OR1/1
  Demux/10 -> Shift Arithmetic2/1
  Bitwise OR4/1 -> Data Type Conversion3/1  "x_axis"
  Demux/9 -> Bitwise OR2/1
  Gain3/1 -> Bias2/1
  Shift Arithmetic6/1 -> Bitwise OR6/2
  Mux2/1 -> Data Type Conversion2/1
  Data Type Conversion3/1 -> Gain3/1
  Bitwise OR2/1 -> Mux2/1  "x_axis"
  Gain1/1 -> acc/1
  Bitwise OR5/1 -> Mux1/1  "x_axis"
  Demux/13 -> Bitwise OR7/1
  Bitwise OR6/1 -> Mux1/2  "x_axis"
  Data Type Conversion1/1 -> Gain6/1
  Shift Arithmetic3/1 -> Bitwise OR3/2
  Cast To Single7/1 -> Demux/1
  Demux/1 -> Bitwise OR4/1
  Demux/12 -> Shift Arithmetic3/1
  Data Type Conversion2/1 -> Gain1/1
  Demux/11 -> Bitwise OR3/1
  Shift Arithmetic4/1 -> Bitwise OR4/2
  Bias2/1 -> Temp/1
  Shift Arithmetic5/1 -> Bitwise OR5/2
  Demux/2 -> Shift Arithmetic4/1
  Demux/5 -> Bitwise OR6/1
  Demux/3 -> Bitwise OR5/1
  Shift Arithmetic7/1 -> Bitwise OR7/2
  Demux/8 -> Shift Arithmetic1/1
  Mux1/1 -> Data Type Conversion1/1
  Demux/14 -> Shift Arithmetic7/1
  Demux/4 -> Shift Arithmetic5/1
  Gain6/1 -> gyro/1
  Bitwise OR3/1 -> Mux2/2  "x_axis"
  Demux/6 -> Shift Arithmetic6/1
  I2C Master Read7/1 -> Cast To Single7/1

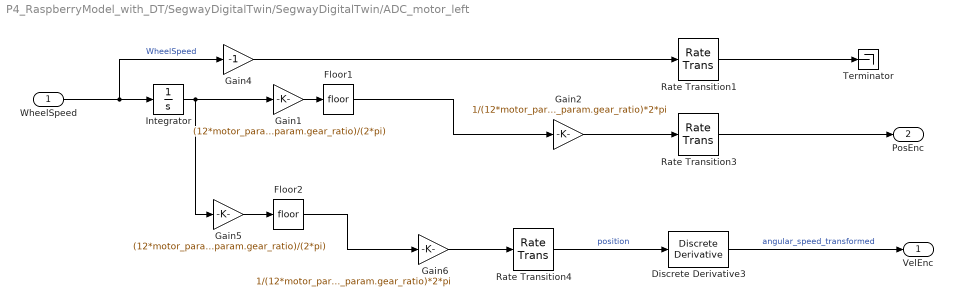
== system P4_RaspberryModel_with_DT/SegwayDigitalTwin/SegwayDigitalTwin/ADC_motor_left ==
  WheelSpeed : Inport
  Discrete Derivative3 : simulink/Discrete/Discrete Derivative  gainval=1  ICPrevScaledInput=0.0  OutMin=[]  OutMax=[]  OutDataType=fixdt(1, 16)  OutScaling=2^-10  DoSatur=off
  Floor1 : Rounding
  Floor2 : Rounding
  Gain1 : Gain  Gain=(12*motor_param.motor_ratio*motor_param.gear_ratio)/(2*pi)
  Gain2 : Gain  Gain=1/(12*motor_param.motor_ratio*motor_param.gear_ratio)*2*pi  OutDataTypeStr=double
  Gain4 : Gain  Gain=-1
  Gain5 : Gain  Gain=(12*motor_param.motor_ratio*motor_param.gear_ratio)/(2*pi)
  Gain6 : Gain  Gain=1/(12*motor_param.motor_ratio*motor_param.gear_ratio)*2*pi  OutDataTypeStr=double
  Integrator : Integrator
  Rate Transition1 : RateTransition  OutPortSampleTime=0.01
  Rate Transition3 : RateTransition  OutPortSampleTime=0.01
  Rate Transition4 : RateTransition  OutPortSampleTime=0.01
  Terminator : Terminator
  VelEnc : Outport
  PosEnc : Outport  Port=2
  wires:
  WheelSpeed/1 -> Integrator/1, Gain4/1  "WheelSpeed"
  Rate Transition3/1 -> PosEnc/1
  Gain2/1 -> Rate Transition3/1
  Floor1/1 -> Gain2/1
  Integrator/1 -> Gain5/1, Gain1/1
  Rate Transition1/1 -> Terminator/1
  Gain4/1 -> Rate Transition1/1
  Discrete Derivative3/1 -> VelEnc/1  "angular_speed_transformed"
  Gain1/1 -> Floor1/1
  Gain5/1 -> Floor2/1
  Floor2/1 -> Gain6/1
  Gain6/1 -> Rate Transition4/1
  Rate Transition4/1 -> Discrete Derivative3/1  "position"

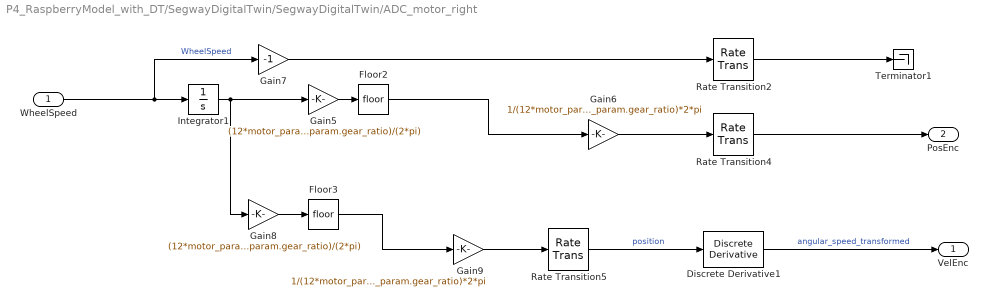
== system P4_RaspberryModel_with_DT/SegwayDigitalTwin/SegwayDigitalTwin/ADC_motor_right ==
  WheelSpeed : Inport
  Discrete Derivative1 : simulink/Discrete/Discrete Derivative  gainval=1  ICPrevScaledInput=0.0  OutMin=[]  OutMax=[]  OutDataType=fixdt(1, 16)  OutScaling=2^-10  DoSatur=off
  Floor2 : Rounding
  Floor3 : Rounding
  Gain5 : Gain  Gain=(12*motor_param.motor_ratio*motor_param.gear_ratio)/(2*pi)
  Gain6 : Gain  Gain=1/(12*motor_param.motor_ratio*motor_param.gear_ratio)*2*pi  OutDataTypeStr=double
  Gain7 : Gain  Gain=-1
  Gain8 : Gain  Gain=(12*motor_param.motor_ratio*motor_param.gear_ratio)/(2*pi)
  Gain9 : Gain  Gain=1/(12*motor_param.motor_ratio*motor_param.gear_ratio)*2*pi  OutDataTypeStr=double
  Integrator1 : Integrator
  Rate Transition2 : RateTransition  OutPortSampleTime=0.01
  Rate Transition4 : RateTransition  OutPortSampleTime=0.01
  Rate Transition5 : RateTransition  OutPortSampleTime=0.01
  Terminator1 : Terminator
  VelEnc : Outport
  PosEnc : Outport  Port=2
  wires:
  Rate Transition2/1 -> Terminator1/1
  Gain9/1 -> Rate Transition5/1
  Floor3/1 -> Gain9/1
  Rate Transition5/1 -> Discrete Derivative1/1  "position"
  Floor2/1 -> Gain6/1
  Rate Transition4/1 -> PosEnc/1
  Gain7/1 -> Rate Transition2/1
  Integrator1/1 -> Gain8/1, Gain5/1
  WheelSpeed/1 -> Integrator1/1, Gain7/1  "WheelSpeed"
  Gain5/1 -> Floor2/1
  Gain8/1 -> Floor3/1
  Discrete Derivative1/1 -> VelEnc/1  "angular_speed_transformed"
  Gain6/1 -> Rate Transition4/1

== system P4_RaspberryModel_with_DT/SegwayDigitalTwin/SegwayDigitalTwin/DAC left ==
  PWM_In : Inport
  Dir_In : Inport  Port=2
  Data Type Conversion : DataTypeConversion  OutDataTypeStr=double  SaturateOnIntegerOverflow=off  RndMeth=Floor
  Data Type Conversion1 : DataTypeConversion  OutDataTypeStr=double  SaturateOnIntegerOverflow=off  RndMeth=Floor
  First Order Hold : FirstOrderHold  ErrorTolerance=inf
  First Order Hold1 : FirstOrderHold  ErrorTolerance=inf
  PWM_Out : Outport
  Dir_Out : Outport  Port=2
  wires:
  Dir_In/1 -> Data Type Conversion1/1
  First Order Hold1/1 -> Dir_Out/1
  First Order Hold/1 -> PWM_Out/1
  Data Type Conversion1/1 -> First Order Hold1/1
  Data Type Conversion/1 -> First Order Hold/1
  PWM_In/1 -> Data Type Conversion/1

== system P4_RaspberryModel_with_DT/SegwayDigitalTwin/SegwayDigitalTwin/DAC right ==
  PWM_In : Inport
  Dir_In : Inport  Port=2
  Data Type Conversion : DataTypeConversion  OutDataTypeStr=double  SaturateOnIntegerOverflow=off  RndMeth=Floor
  Data Type Conversion1 : DataTypeConversion  OutDataTypeStr=double  SaturateOnIntegerOverflow=off  RndMeth=Floor
  First Order Hold : FirstOrderHold  ErrorTolerance=inf
  First Order Hold1 : FirstOrderHold  ErrorTolerance=inf
  PWM_Out : Outport
  Dir_Out : Outport  Port=2
  wires:
  PWM_In/1 -> Data Type Conversion/1
  Data Type Conversion/1 -> First Order Hold/1
  Data Type Conversion1/1 -> First Order Hold1/1
  First Order Hold/1 -> PWM_Out/1
  First Order Hold1/1 -> Dir_Out/1
  Dir_In/1 -> Data Type Conversion1/1

== system P4_RaspberryModel_with_DT/SegwayDigitalTwin/SegwayDigitalTwin/Motor Control left ==
  In1 : Inport
  In2 : Inport  Port=2
  Abs1 : Abs  SaturateOnIntegerOverflow=off  OutDataTypeStr=Inherit: Inherit via internal rule
  Compare To Zero1 : simulink/Logic and Bit Operations/Compare To Zero  relop=<=  OutDataTypeStr=boolean
  PID Controller : slpidlib/PID Controller  Controller=PID  Form=Parallel  TimeDomain=Discrete-time  UseExternalTs=off  SampleTime=0.01  IntegratorMethod=Forward Euler  FilterMethod=Forward Euler  ControllerParametersSource=internal  P=motor_left.P  I=motor_left.I  UseKiTs=off  D=motor_left.D  UseExternalDerivativeSource=off  N=motor_left.N  UseFilter=on  TunerSelectOption=Transfer Function Based (PID Tuner App)  InitialConditionSource=internal  InitialConditionForIntegrator=0  InitialConditionForFilter=0  DifferentiatorICPrevScaledInput=0  ExternalReset=none  TrackingMode=off  Kt=1  LimitOutput=on  SatLimitsSource=internal  UpperSaturationLimit=250  LowerSaturationLimit=-250  LinearizeAsGain=on  AntiWindupMode=back-calculation  Kb=1  LimitIntegrator=off  UpperIntegratorSaturationLimit=inf  LowerIntegratorSaturationLimit=-inf  POutMin=[]  POutMax=[]  IOutMin=[]  IOutMax=[]  DOutMin=[]  DOutMax=[]  NOutMin=[]  NOutMax=[]  SumOutMin=[]  SumOutMax=[]  SaturationOutMin=[]  SaturationOutMax=[]  PParamMin=[]  PParamMax=[]  IParamMin=[]  IParamMax=[]  DParamMin=[]  DParamMax=[]  NParamMin=[]  NParamMax=[]  KbParamMin=[]  KbParamMax=[]  KtParamMin=[]  KtParamMax=[]  KbOutMin=[]  KbOutMax=[]  KtOutMin=[]  KtOutMax=[]  IntegratorOutMin=[]  IntegratorOutMax=[]  FilterOutMin=[]  FilterOutMax=[]  SumI1OutMin=[]  SumI1OutMax=[]  SumI2OutMin=[]  SumI2OutMax=[]  SumI3OutMin=[]  SumI3OutMax=[]  SumI4OutMin=[]  SumI4OutMax=[]  SumDOutMin=[]  SumDOutMax=[]  DifferentiatorOutMin=[]  DifferentiatorOutMax=[]  FilterDiffOutCoefMin=[]  FilterDiffOutCoefMax=[]  ReciprocalOutMin=[]  ReciprocalOutMax=[]  SumDenOutMin=[]  SumDenOutMax=[]  SumNumOutMin=[]  SumNumOutMax=[]  DivideOutMin=[]  DivideOutMax=[]  UdiffTsProdOutMin=[]  UdiffTsProdOutMax=[]  NTsProdOutMin=[]  NTsProdOutMax=[]  UintegralTsProdOutMin=[]  UintegralTsProdOutMax=[]  UngainTsProdOutMin=[]  UngainTsProdOutMax=[]  ClampingZeroOutDataTypeStr=Inherit: Inherit via back propagation  ClampingZeroOutMin=[]  ClampingZeroOutMax=[]  FilterDenConstantOutDataTypeStr=Inherit: Inherit via back propagation  FilterDenConstantOutMin=[]  FilterDenConstantOutMax=[]  PCopyOutDataTypeStr=Inherit: Inherit via back propagation  PCopyOutMin=[]  PCopyOutMax=[]  NCopyOutDataTypeStr=Inherit: Inherit via back propagation  NCopyOutMin=[]  NCopyOutMax=[]  IntegratorContinuousStateAttributes=''  IntegratorStateMustResolveToSignalObject=off  IntegratorRTWStateStorageClass=Auto  FilterContinuousStateAttributes=''  FilterStateMustResolveToSignalObject=off  FilterRTWStateStorageClass=Auto  ParallelPVariant=InternalParameters  IdealPVariant=Disabled  IVariant=InternalParameters  DVariant=InternalParameters  IntegratorVariant=Discrete  SatVariant=Enabled  AWVariant=BackCalculation  PCopyVariant=Disabled  TRVariant=Disabled  FdbkBlocksVariant=Forward  IdealPFdbkVariant=Disabled  SatFdbkVariant=Disabled  DerivativeFilterVariant=ForwardEulerFilter  NVariant=InternalParameters  NCopyVariant=Disabled  FilterICVariant=InternalICsFilter  IntegratorICVariant=InternalICs  ExternalResetVariant=Disabled  TRSumVariant=Passthrough  SumFdbkVariant=Disabled  SumVariant=Sum_PID  TsampFilterVariant=InternalTs  TsampNgainVariant=Passthrough  TsampIntegralVariant=Disabled_SignalSpec  ExternalSaturationOutDataTypeStr=Inherit: Same as second input  DerivativeSourceVariant=ErrorSignal  PreIntVariant=InternalPreInt
  Subtract : Sum  Inputs=+-|
  PWMDutyCycle : Outport
  RevolutionDirection : Outport  Port=2
  wires:
  In1/1 -> Subtract/1
  In2/1 -> Subtract/2
  Subtract/1 -> PID Controller/1  "SpeedError"
  Compare To Zero1/1 -> RevolutionDirection/1  "RevolutionDirection"
  PID Controller/1 -> Compare To Zero1/1, Abs1/1  "SpeedControllerOutput"
  Abs1/1 -> PWMDutyCycle/1  "PWMDutyCycle"

== system P4_RaspberryModel_with_DT/SegwayDigitalTwin/SegwayDigitalTwin/Motor Control right ==
  In1 : Inport
  In2 : Inport  Port=2
  Abs1 : Abs  SaturateOnIntegerOverflow=off  OutDataTypeStr=Inherit: Inherit via internal rule
  Compare To Zero1 : simulink/Logic and Bit Operations/Compare To Zero  relop=<=  OutDataTypeStr=boolean
  PID Controller : slpidlib/PID Controller  Controller=PID  Form=Parallel  TimeDomain=Discrete-time  UseExternalTs=off  SampleTime=0.01  IntegratorMethod=Forward Euler  FilterMethod=Forward Euler  ControllerParametersSource=internal  P=motor_right.P  I=motor_right.I  UseKiTs=off  D=motor_right.D  UseExternalDerivativeSource=off  N=motor_right.N  UseFilter=on  TunerSelectOption=Transfer Function Based (PID Tuner App)  InitialConditionSource=internal  InitialConditionForIntegrator=0  InitialConditionForFilter=0  DifferentiatorICPrevScaledInput=0  ExternalReset=none  TrackingMode=off  Kt=1  LimitOutput=on  SatLimitsSource=internal  UpperSaturationLimit=250  LowerSaturationLimit=-250  LinearizeAsGain=on  AntiWindupMode=clamping  Kb=1  LimitIntegrator=off  UpperIntegratorSaturationLimit=250  LowerIntegratorSaturationLimit=-250  POutMin=[]  POutMax=[]  IOutMin=[]  IOutMax=[]  DOutMin=[]  DOutMax=[]  NOutMin=[]  NOutMax=[]  SumOutMin=[]  SumOutMax=[]  SaturationOutMin=[]  SaturationOutMax=[]  PParamMin=[]  PParamMax=[]  IParamMin=[]  IParamMax=[]  DParamMin=[]  DParamMax=[]  NParamMin=[]  NParamMax=[]  KbParamMin=[]  KbParamMax=[]  KtParamMin=[]  KtParamMax=[]  KbOutMin=[]  KbOutMax=[]  KtOutMin=[]  KtOutMax=[]  IntegratorOutMin=[]  IntegratorOutMax=[]  FilterOutMin=[]  FilterOutMax=[]  SumI1OutMin=[]  SumI1OutMax=[]  SumI2OutMin=[]  SumI2OutMax=[]  SumI3OutMin=[]  SumI3OutMax=[]  SumI4OutMin=[]  SumI4OutMax=[]  SumDOutMin=[]  SumDOutMax=[]  DifferentiatorOutMin=[]  DifferentiatorOutMax=[]  FilterDiffOutCoefMin=[]  FilterDiffOutCoefMax=[]  ReciprocalOutMin=[]  ReciprocalOutMax=[]  SumDenOutMin=[]  SumDenOutMax=[]  SumNumOutMin=[]  SumNumOutMax=[]  DivideOutMin=[]  DivideOutMax=[]  UdiffTsProdOutMin=[]  UdiffTsProdOutMax=[]  NTsProdOutMin=[]  NTsProdOutMax=[]  UintegralTsProdOutMin=[]  UintegralTsProdOutMax=[]  UngainTsProdOutMin=[]  UngainTsProdOutMax=[]  ClampingZeroOutDataTypeStr=Inherit: Inherit via back propagation  ClampingZeroOutMin=[]  ClampingZeroOutMax=[]  FilterDenConstantOutDataTypeStr=Inherit: Inherit via back propagation  FilterDenConstantOutMin=[]  FilterDenConstantOutMax=[]  PCopyOutDataTypeStr=Inherit: Inherit via back propagation  PCopyOutMin=[]  PCopyOutMax=[]  NCopyOutDataTypeStr=Inherit: Inherit via back propagation  NCopyOutMin=[]  NCopyOutMax=[]  IntegratorContinuousStateAttributes=''  IntegratorStateMustResolveToSignalObject=off  IntegratorRTWStateStorageClass=Auto  FilterContinuousStateAttributes=''  FilterStateMustResolveToSignalObject=off  FilterRTWStateStorageClass=Auto  ParallelPVariant=InternalParameters  IdealPVariant=Disabled  IVariant=InternalParameters  DVariant=InternalParameters  IntegratorVariant=Discrete  SatVariant=Enabled  AWVariant=DiscClampingParallel  PCopyVariant=Disabled  TRVariant=Disabled  FdbkBlocksVariant=Forward  IdealPFdbkVariant=Disabled  SatFdbkVariant=Disabled  DerivativeFilterVariant=ForwardEulerFilter  NVariant=InternalParameters  NCopyVariant=Disabled  FilterICVariant=InternalICsFilter  IntegratorICVariant=InternalICs  ExternalResetVariant=Disabled  TRSumVariant=Passthrough  SumFdbkVariant=Disabled  SumVariant=Sum_PID  TsampFilterVariant=InternalTs  TsampNgainVariant=Passthrough  TsampIntegralVariant=Disabled_SignalSpec  ExternalSaturationOutDataTypeStr=Inherit: Same as second input  DerivativeSourceVariant=ErrorSignal  PreIntVariant=InternalPreInt
  Subtract : Sum  Inputs=+-|
  PWMDutyCycle : Outport
  RevolutionDirection : Outport  Port=2
  wires:
  In1/1 -> Subtract/1
  In2/1 -> Subtract/2
  Subtract/1 -> PID Controller/1  "SpeedError"
  Compare To Zero1/1 -> RevolutionDirection/1  "RevolutionDirection"
  PID Controller/1 -> Compare To Zero1/1, Abs1/1  "SpeedControllerOutput"
  Abs1/1 -> PWMDutyCycle/1  "PWMDutyCycle"

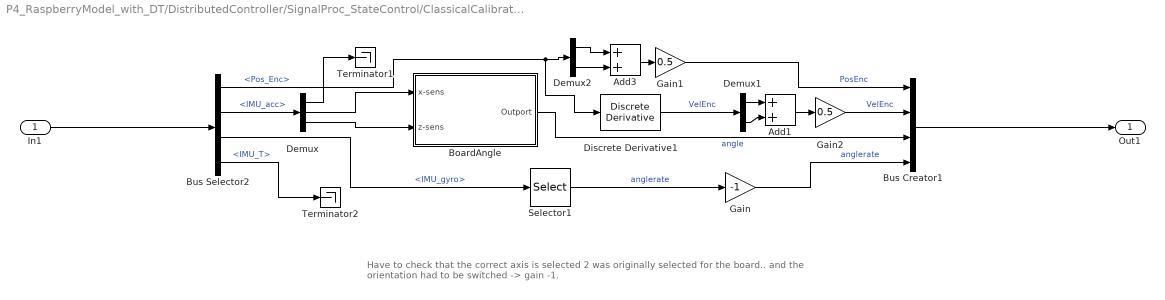
== system P4_RaspberryModel_with_DT/DistributedController/SignalProc_StateControl/ClassicalCalibration/SensorProcessing ==
  note: Have to check that the correct axis is selected 2 was originally selected for the board.. and the orientation had to be switched -> gain -1.
  In1 : Inport
  Add1 : Sum
  Add3 : Sum
  BoardAngle : Subsystem
  Bus Creator1 : BusCreator  Inputs=4  OutDataTypeStr=Bus: States
  Bus Selector2 : BusSelector  OutputSignals=Pos_Enc,IMU_acc,IMU_gyro,IMU_T
  Demux : Demux  Outputs=3
  Demux1 : Demux  Outputs=2
  Demux2 : Demux  Outputs=2
  Discrete Derivative1 : simulink/Discrete/Discrete Derivative  gainval=1.0  ICPrevScaledInput=0.0  OutMin=[]  OutMax=[]  OutDataType=fixdt(1, 16)  OutScaling=2^-10  DoSatur=off
  Gain : Gain  Gain=-1
  Gain1 : Gain  Gain=0.5
  Gain2 : Gain  Gain=0.5
  Selector1 : Selector  InputPortWidth=3  IndexOptions=Index vector (dialog)  Indices=[1]  OutputSizes=1
  Terminator1 : Terminator
  Terminator2 : Terminator
  Out1 : Outport  OutDataTypeStr=Bus: States
  wires:
  Bus Selector2/3 -> Selector1/1  "<IMU_gyro>"
  Add3/1 -> Gain1/1
  Bus Selector2/2 -> Demux/1  "<IMU_acc>"
  Demux/1 -> Terminator1/1
  Selector1/1 -> Gain/1  "anglerate"
  Bus Selector2/4 -> Terminator2/1  "<IMU_T>"
  Bus Selector2/1 -> Discrete Derivative1/1, Demux2/1  "<Pos_Enc>"
  Demux/3 -> BoardAngle/2(z-sens)
  Discrete Derivative1/1 -> Demux1/1  "VelEnc"
  Demux2/2 -> Add3/2
  Gain1/1 -> Bus Creator1/1  "PosEnc"
  BoardAngle/1(Outport) -> Bus Creator1/3  "angle"
  Demux2/1 -> Add3/1
  Bus Creator1/1 -> Out1/1
  In1/1 -> Bus Selector2/1
  Demux1/2 -> Add1/2
  Demux1/1 -> Add1/1
  Add1/1 -> Gain2/1
  Gain2/1 -> Bus Creator1/2  "VelEnc"
  Gain/1 -> Bus Creator1/4  "anglerate"
  Demux/2 -> BoardAngle/1(x-sens)

== system P4_RaspberryModel_with_DT/DistributedController/SignalProc_StateControl/ClassicalCalibration/Statemachine_Old ==
  In1 : Inport
  setpoint : Inport  Port=2
  Add : Sum  Inputs=+-
  Bus Creator : BusCreator  Inputs=4
  Bus Selector1 : BusSelector  OutputSignals=PosEnc,VelEnc,angle,anglerate
  StateControl : Subsystem
  Terminator : Terminator
  SigiState : Outport  OutDataTypeStr=Bus: States
  pos_error : Outport  Port=2
  active : Outport  Port=3
  wires:
  StateControl/2(velocity) -> Bus Creator/2  "VelEnc"
  Bus Selector1/3 -> StateControl/3(Acc)  "<angle>"
  Bus Selector1/2 -> StateControl/2(VelEnc)  "<VelEnc>"
  Bus Selector1/4 -> StateControl/4(Gyro)  "<anglerate>"
  StateControl/4(anglerate) -> Bus Creator/4  "anglerate"
  Bus Selector1/1 -> StateControl/1(PosEnc)  "<PosEnc>"
  StateControl/1(position) -> Bus Creator/1, Add/2  "PosEnc"
  StateControl/6(state) -> Terminator/1
  StateControl/3(angle) -> Bus Creator/3  "angle"
  In1/1 -> Bus Selector1/1
  Bus Creator/1 -> SigiState/1
  StateControl/5(active) -> active/1
  setpoint/1 -> Add/1
  Add/1 -> pos_error/1
